simulink model "model_upwind"  (R2020b)
settings: Solver=VariableStepAuto  StartTime=0.0  StopTime=10.0  RelTol=1e-3
undefined symbols (not defined in the file or in its folder): upwind, upwind_height_end, upwind_height_start, upwind_lat_end, upwind_lat_start, upwind_lon_end, upwind_lon_start
settings Model: Creator=C:\Users\Dogukan  LastModifiedBy=C:\Users\Dogukan

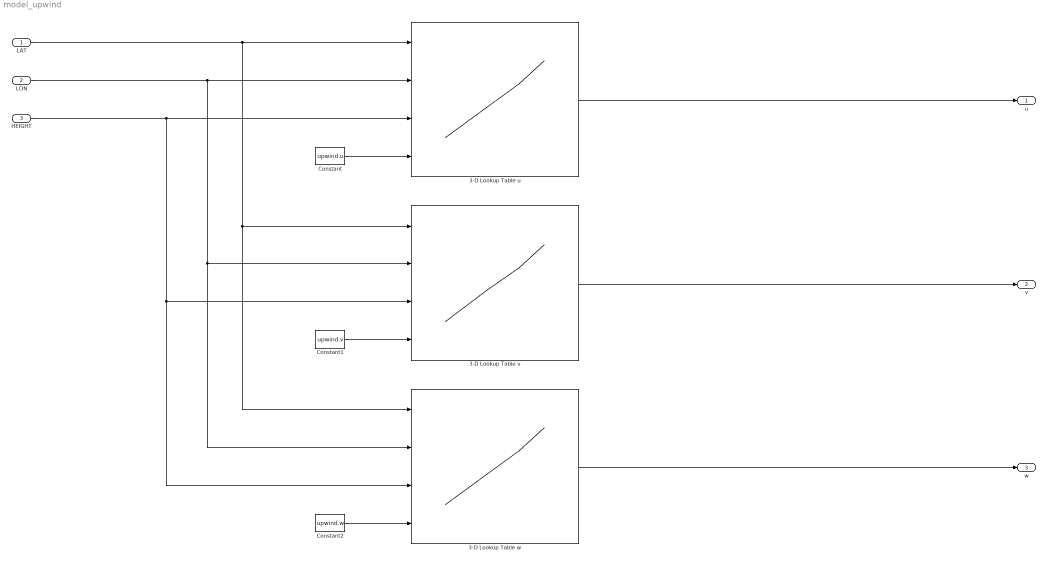
== system model_upwind ==
  LAT : Inport
  LON : Inport  Port=2
  HEIGHT : Inport  Port=3
  3-D Lookup Table u : Lookup_n-D  NumberOfTableDimensions=3  BreakpointsForDimension1=linspace(upwind_lat_start, upwind_lat_end, 100)  BreakpointsForDimension2=linspace(upwind_lon_start, upwind_lon_end, 100)  BreakpointsForDimension3=linspace(upwind_height_start, upwind_height_end, 100)  TableSource=Input port  Table=reshape(repmat([4 5 6;16 19 20;10 18 23],1,2),[3,3,2])  ExtrapMethod=Clip  InternalRulePriority=Speed  RndMeth=Simplest  InputSameDT=on
      settings: InputPortMap=u0,u1,u2,p221
  3-D Lookup Table v : Lookup_n-D  NumberOfTableDimensions=3  BreakpointsForDimension1=linspace(upwind_lat_start, upwind_lat_end, 100)  BreakpointsForDimension2=linspace(upwind_lon_start, upwind_lon_end, 100)  BreakpointsForDimension3=linspace(upwind_height_start, upwind_height_end, 100)  TableSource=Input port  Table=reshape(repmat([4 5 6;16 19 20;10 18 23],1,2),[3,3,2])  ExtrapMethod=Clip  InternalRulePriority=Speed  RndMeth=Simplest  InputSameDT=on
      settings: InputPortMap=u0,u1,u2,p221
  3-D Lookup Table w : Lookup_n-D  NumberOfTableDimensions=3  BreakpointsForDimension1=linspace(upwind_lat_start, upwind_lat_end, 100)  BreakpointsForDimension2=linspace(upwind_lon_start, upwind_lon_end, 100)  BreakpointsForDimension3=linspace(upwind_height_start, upwind_height_end, 100)  TableSource=Input port  Table=reshape(repmat([4 5 6;16 19 20;10 18 23],1,2),[3,3,2])  ExtrapMethod=Clip  InternalRulePriority=Speed  RndMeth=Simplest  InputSameDT=on
      settings: InputPortMap=u0,u1,u2,p221
  Constant : Constant  Value=upwind.u
  Constant1 : Constant  Value=upwind.v
  Constant2 : Constant  Value=upwind.w
  u : Outport
  v : Outport  Port=2
  w : Outport  Port=3
  wires:
  LAT/1 -> 3-D Lookup Table u/1, 3-D Lookup Table v/1, 3-D Lookup Table w/1
  LON/1 -> 3-D Lookup Table w/2, 3-D Lookup Table v/2, 3-D Lookup Table u/2
  HEIGHT/1 -> 3-D Lookup Table w/3, 3-D Lookup Table v/3, 3-D Lookup Table u/3
  3-D Lookup Table w/1 -> w/1
  3-D Lookup Table v/1 -> v/1
  3-D Lookup Table u/1 -> u/1
  Constant/1 -> 3-D Lookup Table u/4
  Constant1/1 -> 3-D Lookup Table v/4
  Constant2/1 -> 3-D Lookup Table w/4
